simulink model "vcrankex"  (Simulink 3.00)
settings: Solver=FixedStepDiscrete  StartTime=0.0  StopTime=10.0  RelTol=1e-3
libraries: smxl x1
settings Model: LastModifiedBy=giampiero

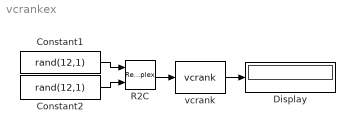
== system vcrankex ==
  Constant1 : Constant  Value=rand(12,1)
  Constant2 : Constant  Value=rand(12,1)
  Display : Display
      settings: Format=short
  R2C : RealImagToComplex  Input=RealAndImag  ConstantPart=0
  vcrank : smxl/Complex Matrices/vcrank  d=[4 3]  tol=1
  wires:
  Constant1/1 -> R2C/1
  Constant2/1 -> R2C/2
  vcrank/1 -> Display/1
  R2C/1 -> vcrank/1
